simulink model "SOC_EKF_estimator_prev"  (R2024a)
settings: configuration reference "BMS_Base_ModelReferencingConfig" (kept outside this file)
values from neighbouring files (symbols this model uses):
  BATTERY_MODULE_CAPACITY_AH = 51.0    [ParametersDataDictionary.sldd]    (also in SOXDictionary.sldd; SOXDictionaryGotion.sldd = 116.0
  ECM_C1_C = 5154.0 7026.0 9772.0 9147.0 5282.0 6834.0 13304.0 9147.0 6022.0 5723.0 19827.0 8949.0 6094.0 5723.0 6902.0 8949.0 4616.0 11831.0 6902.0 13350.0 5313.0 9929.0 17487.0 13353.0 8639.0 11887.0 9132.0 11502.0 6626.0 7280.0 9137.0 5520.0 9337.0 7280.0 11758.0 5511.0 9338.0 6268.0 11758.0 9195.0 6039.0 6263.0 20048.0 9182.0 6046.0 6328.0 12260.0 8896.0 6354.0 6473.0 18161.0 9934.0 6987.0 6000.0 9292.0 15    [ParametersDataDictionary.sldd]    (also in SOXDictionary.sldd; SOXDictionaryGotion.sldd = 9377.3935549443049 12784.352117101025 17780.50497472 16643.1)
  ECM_C1_D = 3228.0 2948.0 5233.0 5436.0 5811.0 4127.0 6804.0 6524.0 8135.0 4952.0 8164.0 7176.0 9961.0 5636.0 7911.0 9532.0 9960.0 9207.0 8366.0 9401.0 8460.0 9396.0 12773.0 9959.0 8460.0 9395.0 12772.0 9964.0 7834.0 10153.0 5968.0 9123.0 6541.0 18964.0 9267.0 8525.0 8123.0 12313.0 8367.0 3742.0 6442.0 12210.0 8366.0 3428.0 5988.0 9558.0 8077.0 8045.0 4643.0 5518.0 7691.0 8540.0 4456.0 5518.0 5995.0 7286.0 62    [ParametersDataDictionary.sldd]    (also in SOXDictionary.sldd; SOXDictionaryGotion.sldd = 5874.2494091340313 5363.6664326091695 9522.8556893689238 989)
  ECM_C2_C = 45772.0 48984.0 24783.0 56515.0 42175.0 48984.0 32749.0 56515.0 36169.0 43595.0 52239.0 56744.0 41340.0 50607.0 59483.0 68212.0 47524.0 55037.0 72508.0 78331.0 48850.0 56691.0 70550.0 78064.0 45431.0 56140.0 67393.0 82065.0 42984.0 53070.0 60478.0 69996.0 41064.0 47628.0 50122.0 54978.0 43682.0 51420.0 49145.0 51819.0 43541.0 54115.0 46983.0 51110.0 39789.0 52300.0 51134.0 66238.0 45918.0 49782.0    [ParametersDataDictionary.sldd]    (also in SOXDictionary.sldd; SOXDictionaryGotion.sldd = 83286.762427651513 89132.1866794698 45094.898404433654 10283)
  ECM_C2_D = 4760.0 6966.0 42821.0 29934.0 14279.0 20899.0 68514.0 47895.0 28557.0 37618.0 95920.0 57474.0 50490.0 57647.0 73073.0 66990.0 59702.0 68813.0 73222.0 80296.0 61545.0 79350.0 86184.0 82074.0 55391.0 86528.0 88192.0 86426.0 53021.0 84807.0 92745.0 83396.0 50650.0 71191.0 71040.0 80634.0 50050.0 57961.0 70293.0 48270.0 38012.0 52076.0 50396.0 43580.0 30401.0 39369.0 50234.0 78082.0 33602.0 41072.0 66    [ParametersDataDictionary.sldd]    (also in SOXDictionary.sldd; SOXDictionaryGotion.sldd = 8660.4321560409171 12676.055410309849 77918.08252980643 5446)
  ECM_C3_C = 537058.0 589124.0 714633.0 1204481.0 541039.0 568254.0 686461.0 1730326.0 547828.0 680683.0 941505.0 2378176.0 839223.0 1607216.0 3290233.0 3006282.0 1000602.0 1251630.0 3006278.0 3472896.0 1184548.0 1483067.0 3218937.0 3636270.0 1028380.0 1436146.0 2223746.0 3355757.0 745536.0 1168882.0 1688371.0 2653844.0 620308.0 824195.0 1301261.0 2084020.0 446818.0 641457.0 922723.0 1739693.0 342589.0 573506.    [ParametersDataDictionary.sldd]    (also in SOXDictionary.sldd; SOXDictionaryGotion.sldd = 977235.776567173 1071975.4393548302 1300351.5011858649 21916)
  ECM_C3_D = 580.0 7054.0 520703.0 278880.0 5803.0 35269.0 1041407.0 501983.0 58029.0 176346.0 1562110.0 702777.0 550952.0 1077867.0 377705.0 1289111.0 473354.0 778552.0 1457119.0 719377.0 437563.0 643625.0 1059730.0 698669.0 497163.0 691708.0 1156803.0 970788.0 517884.0 785936.0 1130538.0 1035732.0 793531.0 1122645.0 1385533.0 1849087.0 1010883.0 1344004.0 1961793.0 2516467.0 1066704.0 1433795.0 2759419.0 340    [ParametersDataDictionary.sldd]    (also in SOXDictionary.sldd; SOXDictionaryGotion.sldd = 1055.9004514656031 12835.215816146119 947476.12402523274 507)
  ECM_R0_C = 0.00214 0.0015 0.00096 0.00066 0.0019 0.00131 0.00093 0.00065 0.00188 0.00129 0.00088 0.00064 0.00186 0.00126 0.00088 0.00063 0.00184 0.00122 0.00087 0.00062 0.00185 0.0012 0.00085 0.00061 0.00182 0.00119 0.00083 0.00061 0.00179 0.00118 0.00083 0.0006 0.0018 0.00119 0.00083 0.0006 0.00175 0.00118 0.00086 0.00061 0.00174 0.00117 0.00083 0.0006 0.00176 0.00116 0.00082 0.00059 0.00173 0.00116 0.00083    [ParametersDataDictionary.sldd]    (also in SOXDictionary.sldd; SOXDictionaryGotion.sldd = 0.0011762548470330098 0.00082374580425955042 0.0005282200468)
  ECM_R0_D = 0.00213 0.00146 0.00098 0.00068 0.00209 0.0014 0.00095 0.00065 0.00205 0.00134 0.00091 0.00064 0.00197 0.00127 0.00087 0.00062 0.00189 0.0012 0.00082 0.00061 0.00176 0.00121 0.00081 0.00061 0.00179 0.0012 0.00082 0.00062 0.00176 0.0012 0.00081 0.0006 0.00174 0.00118 0.00081 0.00059 0.00173 0.00115 0.0008 0.0006 0.00177 0.00118 0.0008 0.0006 0.0018 0.00118 0.00081 0.0006 0.00184 0.00119 0.0008 0.00    [ParametersDataDictionary.sldd]    (also in SOXDictionary.sldd; SOXDictionaryGotion.sldd = 0.0011713156680267826 0.00080379131757867114 0.0005358497183)
  ECM_R1_C = 0.00086 0.00196 0.00025 0.00099 0.00084 0.00121 0.00025 0.00034 0.00076 0.0009 0.00038 0.00034 0.00076 0.0009 0.00066 0.00034 0.00056 0.00037 0.00066 0.00022 0.00054 0.00033 0.00028 0.00022 0.00039 0.00032 0.0003 0.00019 0.00064 0.00062 0.0003 0.00021 0.0008 0.00062 0.00022 0.00027 0.0008 0.00061 0.00022 0.00031 0.00084 0.00062 0.00023 0.00032 0.00084 0.00058 0.00028 0.00036 0.00076 0.00035 0.0002    [ParametersDataDictionary.sldd]    (also in SOXDictionary.sldd; SOXDictionaryGotion.sldd = 0.00046991497657839924 0.0010779816764740048 0.0001372074802)
  ECM_R1_D = 0.00113 0.00161 0.00086 0.00055 0.00063 0.00115 0.00066 0.00046 0.00045 0.00096 0.00055 0.00042 0.00041 0.00087 0.0005 0.0004 0.00041 0.00055 0.00031 0.00042 0.0004 0.0003 0.00024 0.00029 0.0004 0.0003 0.00024 0.00036 0.00042 0.00038 0.00023 0.00046 0.00049 0.00034 0.00028 0.00048 0.00053 0.00033 0.00045 0.00036 0.00053 0.00034 0.00045 0.00036 0.00079 0.00048 0.00025 0.00028 0.00058 0.0009 0.00045    [ParametersDataDictionary.sldd]    (also in SOXDictionary.sldd; SOXDictionaryGotion.sldd = 0.00062343910396692745 0.00088344565476029683 0.000473998175)
  ECM_R2_C = 0.00238 0.0021 0.00172 0.00051 0.00206 0.00146 0.00107 0.00073 0.00176 0.0013 0.00091 0.0004 0.00156 0.00124 0.00089 0.0004 0.0015 0.00103 0.00083 0.00056 0.00147 0.00104 0.00083 0.00057 0.00152 0.00109 0.00082 0.00053 0.00173 0.00119 0.00091 0.00057 0.00199 0.00148 0.00107 0.00071 0.00214 0.00168 0.00128 0.00087 0.00209 0.00184 0.00138 0.00092 0.00193 0.00149 0.00089 0.00055 0.00164 0.00115 0.000    [ParametersDataDictionary.sldd]    (also in SOXDictionary.sldd; SOXDictionaryGotion.sldd = 0.0013071970907491625 0.0011565350014947392 0.00094770363400)
  ECM_R2_D = 0.01493 0.00869 0.00246 0.0013 0.00498 0.0029 0.00154 0.00082 0.00249 0.00161 0.0011 0.00068 0.00166 0.00134 0.00092 0.00065 0.00169 0.00137 0.00096 0.00066 0.00172 0.00136 0.00106 0.00071 0.00163 0.00129 0.00104 0.00071 0.00161 0.00121 0.00091 0.0006 0.00151 0.0011 0.00076 0.00046 0.0015 0.00107 0.00076 0.00051 0.00158 0.00108 0.00087 0.0006 0.00203 0.00162 0.00094 0.00095 0.00203 0.00165 0.00141    [ParametersDataDictionary.sldd]    (also in SOXDictionary.sldd; SOXDictionaryGotion.sldd = 0.0082023616629522487 0.00477357645651923 0.0013535754139770)
  ECM_R3_C = 0.00415 0.00139 0.00228 0.00107 0.00223 0.00139 0.00065 0.00138 0.00203 0.00126 0.00065 0.00172 0.00121 0.00085 0.00061 0.00132 0.00106 0.00068 0.00039 0.00079 0.00105 0.00069 0.00041 0.00067 0.00113 0.00082 0.00052 0.00037 0.00126 0.00085 0.00052 0.00034 0.00132 0.00102 0.00056 0.00036 0.00183 0.0012 0.00069 0.00041 0.00189 0.00152 0.00079 0.00043 0.0016 0.00126 0.00073 0.00076 0.00138 0.00116 0.    [ParametersDataDictionary.sldd]    (also in SOXDictionary.sldd; SOXDictionaryGotion.sldd = 0.0022791079484232404 0.00076358338365525792 0.0012549156736)
  ECM_R3_D = 1.08481 0.08984 0.00314 0.00567 0.10848 0.01797 0.00157 0.00315 0.01085 0.00359 0.00105 0.00225 0.00181 0.0012 0.0008 0.00204 0.00242 0.00176 0.0008 0.00242 0.00392 0.00242 0.00101 0.00163 0.00237 0.00169 0.00092 0.00071 0.00202 0.00133 0.00067 0.00057 0.00141 0.001 0.00054 0.00038 0.00129 0.00094 0.00048 0.00035 0.00132 0.00103 0.00061 0.00061 0.00401 0.00297 0.00071 0.00075 0.0065 0.00342 0.0008    [ParametersDataDictionary.sldd]    (also in SOXDictionary.sldd; SOXDictionaryGotion.sldd = 0.5961801788597515 0.049373498218042031 0.001723106855668819)
  ECM_SOC : value not decoded    [CellDictionary.sldd]
  ECM_T : value not decoded    [CellDictionary.sldd]
  OCV_SOC : value not decoded    [CellDictionary.sldd]
  OCV_T : value not decoded    [CellDictionary.sldd]
  OCV_V = 3.089975 3.1958025155770748 3.2700856729308603 3.3269062967469782 3.3701558672655878 3.3935018471075473 3.4031249999999997 3.4106750000000003 3.417975 3.4255687342956502 3.4340073517474323 3.44463535689108 3.4571649659479133 3.4695529273207848 3.481325 3.49315 3.5048949462107366 3.5157966467267432 3.5254768755401917 3.534725 3.543897510782176 3.5528756373568848 3.5611426187731481 3.5686 3.575725 3    [CellDictionary.sldd]    (also in Gotion116CellDictionary.sldd; ParametersDataDictionary.sldd = 3.426 3.511 3.595 3.627 3.656 3.705 3.785 3.893 3.955 4.054 ; SOXDictionary.sldd = 3.426 3.511 3.595 3.627 3.656 3.705 3.785 3.893 3.955 4.054 ; SOXDictionaryGotion.sldd = 2.8 3.089975 3.1958025155770748 3.2700856729308603 3.3269062)
  SOC_ESTIM_INIT = 0.5    [ParametersDataDictionary.sldd]    (also in SOXDictionary.sldd = 0.5
  SOC_INITIAL_COVARIANCE : value not decoded    [ParametersDataDictionary.sldd]
  SOC_MEASUREMENT_COVARIANCE = 0.01    [ParametersDataDictionary.sldd]    (also in SOXDictionary.sldd = 0.01
  SOC_STATE_COVARIANCE : value not decoded    [ParametersDataDictionary.sldd]
  SOC_TIMESTEP = 1.0    [SOXDictionary.sldd]    (also in SOXDictionaryGotion.sldd = 1.0
  TOTAL_N_CELL_VOLTAGE = 24    [SOXDictionary.sldd]
  X_INIT : value not decoded    [SOXDictionary.sldd]
settings Model: DataDictionary=BcuModel.sldd  SimulationMode=accelerator  Creator=mmackenzie  LastModifiedBy=jgavidia
settings ConfigSetRef: SourceName=BMS_Base_ModelReferencingConfig

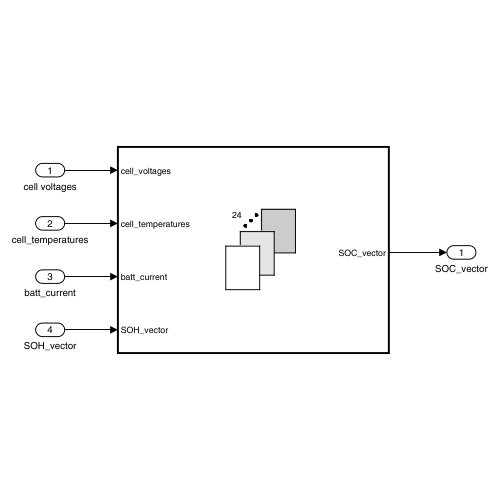
[thumbnail: Simulink's stored preview of the top-level diagram]
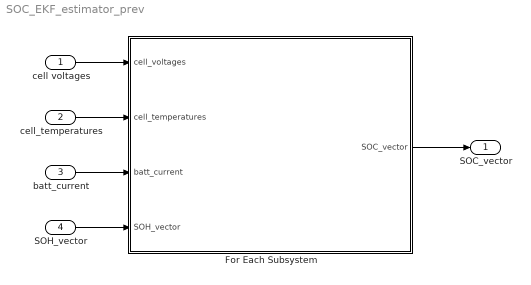
== system SOC_EKF_estimator_prev ==
  cell voltages : Inport  OutDataTypeStr=uint16  PortDimensions=[TOTAL_N_CELL_VOLTAGE,1]
  cell_temperatures : Inport  Port=2  OutDataTypeStr=int16  PortDimensions=[TOTAL_N_CELL_VOLTAGE,1]
  batt_current : Inport  Port=3  OutDataTypeStr=int32  PortDimensions=1
  SOH_vector : Inport  Port=4  OutDataTypeStr=uint16  PortDimensions=[TOTAL_N_CELL_VOLTAGE,1]
  For Each Subsystem : Subsystem  TreatAsAtomicUnit=on
  SOC_vector : Outport  OutDataTypeStr=uint16  PortDimensions=[TOTAL_N_CELL_VOLTAGE,1]
  wires:
  batt_current/1 -> For Each Subsystem/3(batt_current)
  cell_temperatures/1 -> For Each Subsystem/2(cell_temperatures)
  SOH_vector/1 -> For Each Subsystem/4(SOH_vector)
  cell voltages/1 -> For Each Subsystem/1(cell_voltages)
  For Each Subsystem/1(SOC_vector) -> SOC_vector/1

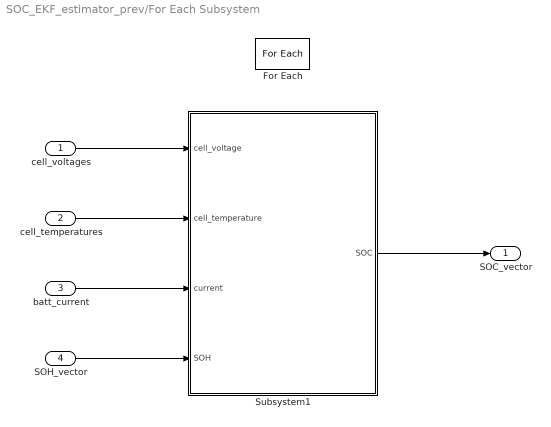
== system SOC_EKF_estimator_prev/For Each Subsystem ==
  cell_voltages : Inport  OutDataTypeStr=uint16  PortDimensions=1  Partition=on  PartitionDimension=1  PartitionWidth=1  PartitionOffset=0
  cell_temperatures : Inport  Port=2  OutDataTypeStr=int16  PortDimensions=1  Partition=on  PartitionDimension=1  PartitionWidth=1  PartitionOffset=0
  batt_current : Inport  Port=3  OutDataTypeStr=int32  PortDimensions=1
  SOH_vector : Inport  Port=4  OutDataTypeStr=uint16  PortDimensions=1  Partition=on  PartitionDimension=1  PartitionWidth=1  PartitionOffset=0
  For Each : ForEach  DisableCoverage=on
  Subsystem1 : Subsystem
  SOC_vector : Outport  OutDataTypeStr=uint16  PortDimensions=1  ConcatenationDimension=1
  wires:
  Subsystem1/1(SOC) -> SOC_vector/1
  cell_voltages/1 -> Subsystem1/1(cell_voltage)
  cell_temperatures/1 -> Subsystem1/2(cell_temperature)
  batt_current/1 -> Subsystem1/3(current)
  SOH_vector/1 -> Subsystem1/4(SOH)

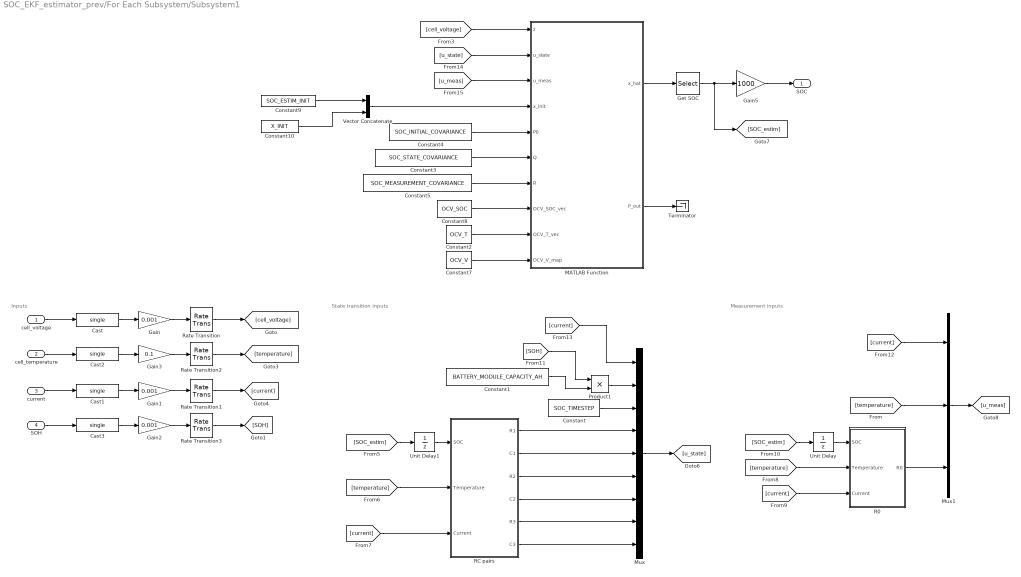
== system SOC_EKF_estimator_prev/For Each Subsystem/Subsystem1 ==
  note: State transition inputs
  note: Inputs
  note: Measurement inputs
  cell_voltage : Inport  OutDataTypeStr=uint16  PortDimensions=1
  cell_temperature : Inport  Port=2  OutDataTypeStr=int16  PortDimensions=1
  current : Inport  Port=3  OutDataTypeStr=int32  PortDimensions=1
  SOH : Inport  Port=4  OutDataTypeStr=uint16  PortDimensions=1
  Cast{,1..3} (4 alike) : DataTypeConversion  OutDataTypeStr=single  SaturateOnIntegerOverflow=off  RndMeth=Floor
  Constant : Constant  Value=SOC_TIMESTEP
  Constant1 : Constant  Value=BATTERY_MODULE_CAPACITY_AH
  Constant10 : Constant  Value=X_INIT  OutDataTypeStr=single
  Constant2 : Constant  Value=OCV_T
  Constant3 : Constant  Value=SOC_STATE_COVARIANCE
  Constant4 : Constant  Value=SOC_INITIAL_COVARIANCE
  Constant5 : Constant  Value=SOC_MEASUREMENT_COVARIANCE
  Constant7 : Constant  Value=OCV_V
  Constant8 : Constant  Value=OCV_SOC
  Constant9 : Constant  Value=SOC_ESTIM_INIT  OutDataTypeStr=single
  Gain : Gain  Gain=0.001
  Gain1 : Gain  Gain=0.001
  Gain2 : Gain  Gain=0.001
  Gain3 : Gain  Gain=0.1
  Gain5 : Gain  Gain=1000  OutDataTypeStr=uint16
  Get SOC : Selector  InputPortWidth=4  IndexOptions=Index vector (dialog)  Indices=1  OutputSizes=1
  MATLAB Function : MATLAB Function  TreatAsAtomicUnit=on
  Mux : Mux  Inputs=9
  Mux1 : Mux  Inputs=3
  Product1 : Product
  R0 : Subsystem
  RC pairs : Subsystem
  Rate Transition{,1..3} (4 alike) : RateTransition  Integrity=off  OutPortSampleTime=1
  Terminator : Terminator
  Unit Delay : UnitDelay  InitialCondition=SOC_ESTIM_INIT  SampleTime=-1  HasFrameUpgradeWarning=on
  Unit Delay1 : UnitDelay  InitialCondition=SOC_ESTIM_INIT  SampleTime=-1  HasFrameUpgradeWarning=on
  Vector Concatenate : Concatenate
  SOC : Outport  OutDataTypeStr=uint16  PortDimensions=1
  wires:
  Gain5/1 -> SOC/1
  Get SOC/1 -> Gain5/1, [SOC_estim]
  Mux1/1 -> [u_meas]
  Constant8/1 -> MATLAB Function/8(OCV_SOC_vec)
  [current] -> Mux1/1
  Cast/1 -> Gain/1
  Cast2/1 -> Gain3/1
  current/1 -> Cast1/1
  [SOC_estim] -> Unit Delay1/1
  [u_state] -> MATLAB Function/2(u_state)
  Constant1/1 -> Product1/2
  MATLAB Function/1(x_hat) -> Get SOC/1
  Gain2/1 -> Rate Transition3/1
  SOH/1 -> Cast3/1
  [temperature] -> R0/2(Temperature)
  Rate Transition/1 -> [cell_voltage]
  Mux/1 -> [u_state]
  Rate Transition1/1 -> [current]
  [current] -> R0/3(Current)
  Gain3/1 -> Rate Transition2/1
  [SOH] -> Product1/1
  Cast1/1 -> Gain1/1
  Constant3/1 -> MATLAB Function/6(Q)
  [temperature] -> Mux1/2
  [temperature] -> RC pairs/2(Temperature)
  Rate Transition2/1 -> [temperature]
  Product1/1 -> Mux/2
  Gain/1 -> Rate Transition/1
  Cast3/1 -> Gain2/1
  cell_voltage/1 -> Cast/1
  Rate Transition3/1 -> [SOH]
  [current] -> Mux/1
  [u_meas] -> MATLAB Function/3(u_meas)
  MATLAB Function/2(P_out) -> Terminator/1
  R0/1(R0) -> Mux1/3
  [cell_voltage] -> MATLAB Function/1(z)
  Unit Delay1/1 -> RC pairs/1(SOC)
  Unit Delay/1 -> R0/1(SOC)
  Constant4/1 -> MATLAB Function/5(P0)
  cell_temperature/1 -> Cast2/1
  Gain1/1 -> Rate Transition1/1
  Constant5/1 -> MATLAB Function/7(R)
  [current] -> RC pairs/3(Current)
  [SOC_estim] -> Unit Delay/1
  RC pairs/1(R1) -> Mux/4
  RC pairs/2(C1) -> Mux/5
  RC pairs/3(R2) -> Mux/6
  RC pairs/4(C2) -> Mux/7
  RC pairs/5(R3) -> Mux/8
  RC pairs/6(C3) -> Mux/9
  Constant/1 -> Mux/3
  Constant2/1 -> MATLAB Function/9(OCV_T_vec)
  Constant7/1 -> MATLAB Function/10(OCV_V_map)
  Constant9/1 -> Vector Concatenate/1
  Constant10/1 -> Vector Concatenate/2
  Vector Concatenate/1 -> MATLAB Function/4(x_init)

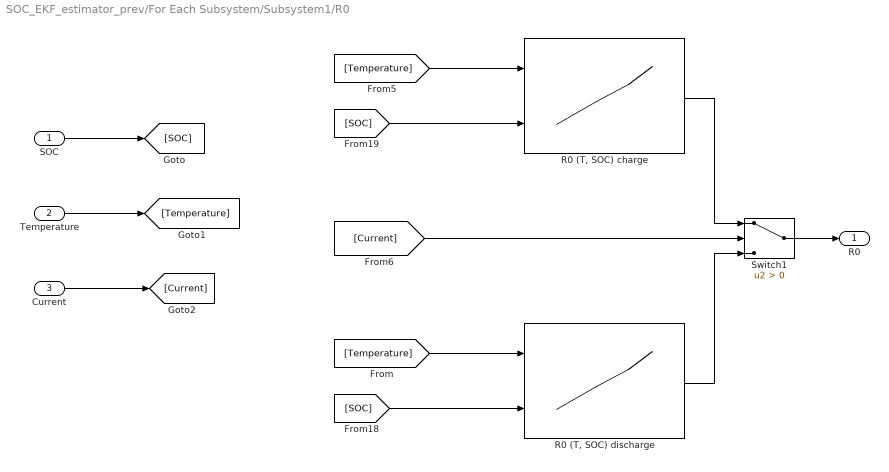
== system SOC_EKF_estimator_prev/For Each Subsystem/Subsystem1/R0 ==
  SOC : Inport
  Temperature : Inport  Port=2
  Current : Inport  Port=3
  "R0 (T, SOC) charge" : Lookup_n-D  BreakpointsForDimension1=ECM_T  BreakpointsForDimension2=ECM_SOC  Table=ECM_R0_C  InternalRulePriority=Speed  RndMeth=Simplest
      settings: InputPortMap=u0,u1
  "R0 (T, SOC) discharge" : Lookup_n-D  BreakpointsForDimension1=ECM_T  BreakpointsForDimension2=ECM_SOC  Table=ECM_R0_D  InternalRulePriority=Speed  RndMeth=Simplest
      settings: InputPortMap=u0,u1
  Switch1 : Switch  Criteria=u2 > Threshold  SaturateOnIntegerOverflow=off  InputSameDT=off
  R0 : Outport
  wires:
  [Temperature] -> "R0 (T, SOC) discharge"/1
  [Current] -> Switch1/2
  Switch1/1 -> R0/1
  Current/1 -> [Current]
  [Temperature] -> "R0 (T, SOC) charge"/1
  SOC/1 -> [SOC]
  [SOC] -> "R0 (T, SOC) charge"/2
  "R0 (T, SOC) discharge"/1 -> Switch1/3
  Temperature/1 -> [Temperature]
  "R0 (T, SOC) charge"/1 -> Switch1/1
  [SOC] -> "R0 (T, SOC) discharge"/2

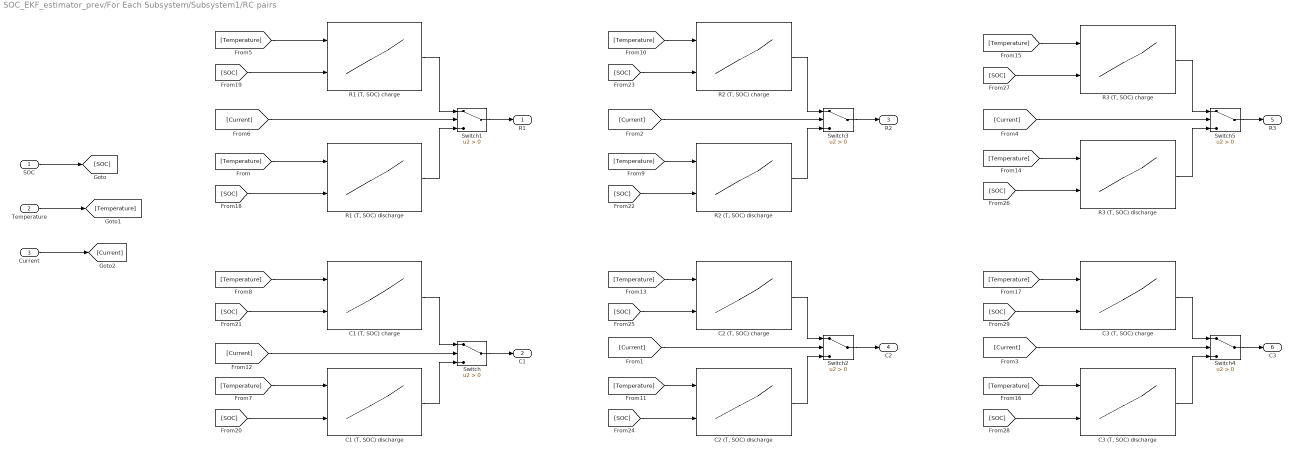
== system SOC_EKF_estimator_prev/For Each Subsystem/Subsystem1/RC pairs ==
  SOC : Inport
  Temperature : Inport  Port=2
  Current : Inport  Port=3
  "C1 (T, SOC) charge" : Lookup_n-D  BreakpointsForDimension1=ECM_T  BreakpointsForDimension2=ECM_SOC  Table=ECM_C1_C  InternalRulePriority=Speed  RndMeth=Simplest
      settings: InputPortMap=u0,u1
  "C1 (T, SOC) discharge" : Lookup_n-D  BreakpointsForDimension1=ECM_T  BreakpointsForDimension2=ECM_SOC  Table=ECM_C1_D  InternalRulePriority=Speed  RndMeth=Simplest
      settings: InputPortMap=u0,u1
  "C2 (T, SOC) charge" : Lookup_n-D  BreakpointsForDimension1=ECM_T  BreakpointsForDimension2=ECM_SOC  Table=ECM_C2_C  InternalRulePriority=Speed  RndMeth=Simplest
      settings: InputPortMap=u0,u1
  "C2 (T, SOC) discharge" : Lookup_n-D  BreakpointsForDimension1=ECM_T  BreakpointsForDimension2=ECM_SOC  Table=ECM_C2_D  InternalRulePriority=Speed  RndMeth=Simplest
      settings: InputPortMap=u0,u1
  "C3 (T, SOC) charge" : Lookup_n-D  BreakpointsForDimension1=ECM_T  BreakpointsForDimension2=ECM_SOC  Table=ECM_C3_C  InternalRulePriority=Speed  RndMeth=Simplest
      settings: InputPortMap=u0,u1
  "C3 (T, SOC) discharge" : Lookup_n-D  BreakpointsForDimension1=ECM_T  BreakpointsForDimension2=ECM_SOC  Table=ECM_C3_D  InternalRulePriority=Speed  RndMeth=Simplest
      settings: InputPortMap=u0,u1
  "R1 (T, SOC) charge" : Lookup_n-D  BreakpointsForDimension1=ECM_T  BreakpointsForDimension2=ECM_SOC  Table=ECM_R1_C  InternalRulePriority=Speed  RndMeth=Simplest
      settings: InputPortMap=u0,u1
  "R1 (T, SOC) discharge" : Lookup_n-D  BreakpointsForDimension1=ECM_T  BreakpointsForDimension2=ECM_SOC  Table=ECM_R1_D  InternalRulePriority=Speed  RndMeth=Simplest
      settings: InputPortMap=u0,u1
  "R2 (T, SOC) charge" : Lookup_n-D  BreakpointsForDimension1=ECM_T  BreakpointsForDimension2=ECM_SOC  Table=ECM_R2_C  InternalRulePriority=Speed  RndMeth=Simplest
      settings: InputPortMap=u0,u1
  "R2 (T, SOC) discharge" : Lookup_n-D  BreakpointsForDimension1=ECM_T  BreakpointsForDimension2=ECM_SOC  Table=ECM_R2_D  InternalRulePriority=Speed  RndMeth=Simplest
      settings: InputPortMap=u0,u1
  "R3 (T, SOC) charge" : Lookup_n-D  BreakpointsForDimension1=ECM_T  BreakpointsForDimension2=ECM_SOC  Table=ECM_R3_C  InternalRulePriority=Speed  RndMeth=Simplest
      settings: InputPortMap=u0,u1
  "R3 (T, SOC) discharge" : Lookup_n-D  BreakpointsForDimension1=ECM_T  BreakpointsForDimension2=ECM_SOC  Table=ECM_R3_D  InternalRulePriority=Speed  RndMeth=Simplest
      settings: InputPortMap=u0,u1
  Switch{,1..5} (6 alike) : Switch  Criteria=u2 > Threshold  SaturateOnIntegerOverflow=off  InputSameDT=off
  R1 : Outport
  C1 : Outport  Port=2
  R2 : Outport  Port=3
  C2 : Outport  Port=4
  R3 : Outport  Port=5
  C3 : Outport  Port=6
  wires:
  Switch1/1 -> R1/1
  Current/1 -> [Current]
  [Current] -> Switch4/2
  "C1 (T, SOC) discharge"/1 -> Switch/3
  [Current] -> Switch1/2
  [SOC] -> "R1 (T, SOC) discharge"/2
  [Current] -> Switch/2
  [SOC] -> "C2 (T, SOC) charge"/2
  SOC/1 -> [SOC]
  [Temperature] -> "R1 (T, SOC) charge"/1
  Switch3/1 -> R2/1
  Switch4/1 -> C3/1
  [SOC] -> "C2 (T, SOC) discharge"/2
  Switch5/1 -> R3/1
  [Temperature] -> "R1 (T, SOC) discharge"/1
  Switch/1 -> C1/1
  [Current] -> Switch3/2
  [SOC] -> "R2 (T, SOC) discharge"/2
  [Temperature] -> "C2 (T, SOC) discharge"/1
  Switch2/1 -> C2/1
  [SOC] -> "R3 (T, SOC) discharge"/2
  "R1 (T, SOC) discharge"/1 -> Switch1/3
  [Temperature] -> "R3 (T, SOC) charge"/1
  "C3 (T, SOC) charge"/1 -> Switch4/1
  [SOC] -> "C1 (T, SOC) discharge"/2
  [Temperature] -> "C3 (T, SOC) charge"/1
  [Temperature] -> "C1 (T, SOC) charge"/1
  [SOC] -> "R3 (T, SOC) charge"/2
  [SOC] -> "R2 (T, SOC) charge"/2
  [SOC] -> "C3 (T, SOC) charge"/2
  "R2 (T, SOC) discharge"/1 -> Switch3/3
  [Temperature] -> "R2 (T, SOC) charge"/1
  "R3 (T, SOC) charge"/1 -> Switch5/1
  [SOC] -> "C1 (T, SOC) charge"/2
  "C2 (T, SOC) charge"/1 -> Switch2/1
  "R2 (T, SOC) charge"/1 -> Switch3/1
  Temperature/1 -> [Temperature]
  [Temperature] -> "R2 (T, SOC) discharge"/1
  "R3 (T, SOC) discharge"/1 -> Switch5/3
  [SOC] -> "C3 (T, SOC) discharge"/2
  [Temperature] -> "C3 (T, SOC) discharge"/1
  [SOC] -> "R1 (T, SOC) charge"/2
  [Temperature] -> "C1 (T, SOC) discharge"/1
  "C2 (T, SOC) discharge"/1 -> Switch2/3
  "C1 (T, SOC) charge"/1 -> Switch/1
  [Temperature] -> "C2 (T, SOC) charge"/1
  [Temperature] -> "R3 (T, SOC) discharge"/1
  [Current] -> Switch5/2
  [Current] -> Switch2/2
  "R1 (T, SOC) charge"/1 -> Switch1/1
  "C3 (T, SOC) discharge"/1 -> Switch4/3

== matlab function SOC_EKF_estimator_prev/For Each Subsystem/Subsystem1/MATLAB Function ==
  data: z input; u_state input; u_meas input; x_init input; P0 input; Q input; R input; OCV_SOC_vec input; x_hat output; P_out output; OCV_T_vec input; OCV_V_map input
function [x_hat, P_out] = EKF_Core(z, u_state, u_meas, x_init, P0, Q, R, OCV_SOC_vec, OCV_T_vec, OCV_V_map)
    % z: Measured voltage (scalar)
    % u_state: [current, capacity, Ts, R1, C1, R2, C2, R3, C3]
    % u_meas: [current, OCV, R0]
    % x_init: initial state estimate [SOC, U1, U2, U3]
    % P0: Initial covariance (4x4 diag matrix)
    % Q: Process noise covariance (4x4 matrix)
    % R: Measurement noise covariance (scalar)
    % OCV_SOC_vec: 1D Vector (e.g., 0:0.1:1)
    % OCV_T_vec: 1D Vector (e.g., [25 35 45])
    % OCV_V_map: 2D Matrix (Rows = SOC, Cols = Temperature)

    % Define persistent variables (the "memory")
    persistent x P
    if isempty(x)
        % Initial State: [SOC; U1; U2; U3]
        x = single(x_init); 
        % Initial Covariance (Uncertainty)
        P = single(P0); 
    end

    % Pre-processing
    curr = u_meas(1); T_cell = u_meas(2); R0 = u_meas(3);
    Ts = u_state(3);
    R1 = u_state(4); C1 = u_state(5);
    R2 = u_state(6); C2 = u_state(7);
    R3 = u_state(8); C3 = u_state(9);

    % --- STEP 1: PREDICT ---
    % Predict the next state using the state transition function
    x_pred = batteryStateTransition(x, u_state);

    % Jacobian A: Linearization of the state transition
    % For RC branches, the derivative is the exponential decay factor
    A = [1, 0,                0, 0;
         0, exp(-Ts/(R1*C1)), 0, 0;
         0, 0, exp(-Ts/(R2*C2)), 0;
         0, 0, 0, exp(-Ts/(R3*C3))];

    P_pred = A * P * A' + Q;

    % --- STEP 2: 2D OCV & SLOPE LOOKUP ---
    % Manually clamp Temperature to the min/max of OCV_T_vec
    T_min = OCV_T_vec(1);
    T_max = OCV_T_vec(end);
    T_clamped = max(T_min, min(T_max, T_cell));

    % Manually clamp SOC to the min/max of OCV_SOC_vec
    SOC_min = OCV_SOC_vec(1);
    SOC_max = OCV_SOC_vec(end);
    soc_clamped = max(SOC_min, min(SOC_max, x_pred(1)));

    % Get OCV at (SOC_pred, T_cell)
    ocv_now = interp2(OCV_T_vec, OCV_SOC_vec, OCV_V_map, T_clamped, soc_clamped, 'linear');

    % Calculate dOCV/dSOC at current temperature
    % Use a small SOC delta to find the local slope on the 2D surface
    eps_soc = 1e-4;
    soc_eps = max(SOC_min, min(SOC_max, soc_clamped + eps_soc));
    ocv_plus = interp2(OCV_T_vec, OCV_SOC_vec, OCV_V_map, T_clamped, soc_eps, 'linear');
    dOCV_dSOC = (ocv_plus - ocv_now) / eps_soc;

    % --- STEP 3: UPDATE ---
    % Predict the measurement (terminal voltage)
    y_pred = ocv_now + x_pred(2) + x_pred(3) + x_pred(4) + (curr * R0);

    % Jacobian H: Linearization of the measurement
    % H = [dOCV/dSOC, dV/dU1, dV/dU2, dV/dU3]
    H = [dOCV_dSOC, 1, 1, 1];

    % Calculate Kalman Gain
    S = H * P_pred * H' + R;       % Innovation covariance
    K = (P_pred * H') / S;         % Kalman Gain

    % Correct the state and covariance based on actual measurement z
    % (JOSEPH FORM UPDATE)
    % Standard P = (I-KH)P can lead to non-positive definite matrices and NaNs.
    % The Joseph form: P = (I - KH)*P_pred*(I - KH)' + K*R*K'
    % is numerically more stable and keeps P symmetric and positive definite.
    I = eye(4);
    x = x_pred + K * (z - y_pred);
    P = (I - K*H) * P_pred * (I - K*H)' + K * R * K';

    % Outputs
    x_hat = x;
    P_out = P;
end

% --- HELPER FUNCTIONS ---

function xNext = batteryStateTransition(x, u)
    current = u(1); capacity = u(2); Ts = u(3);
    R1 = u(4); C1 = u(5); R2 = u(6); C2 = u(7); R3 = u(8); C3 = u(9);

    xdot = zeros(4, 1);
    xdot(1) = current / (3600 * capacity);
    xdot(2) = -1 / (R1 * C1) * x(2) + current / C1;
    xdot(3) = -1 / (R2 * C2) * x(3) + current / C2;
    xdot(4) = -1 / (R3 * C3) * x(4) + current / C3;

    xNext = x + xdot * Ts;
end
